simulink model "system2"  (R2020a)
settings: Solver=ode45  StartTime=0.0  StopTime=1  RelTol=1e-3  EnableMultiTasking=on
libraries: powerlib x76, powerlib_meascontrol x8, simulink_extras x8, re_lib x4
settings Model: Creator=srish  LastModifiedBy=srishtik
settings SolverCC: DecoupledContinuousIntegration=on
settings DataIOCC: LimitDataPoints=on  SaveFormat=Array
settings OptimizationCC: LifeSpan=inf
settings DebuggingCC: ReadBeforeWriteMsg=DisableAll  WriteAfterWriteMsg=DisableAll  WriteAfterReadMsg=DisableAll  SolverPrmCheckMsg=warning  MultiTaskDSMMsg=none  SFUnexpectedBacktrackingDiag=warning  SFNoUnconditionalDefaultTransitionDiag=warning  SFExecutionAtInitializationDiag=none  ArithmeticOperatorsInVariantConditions=warning
settings HardwareCC: ProdBitPerPointer=32  ProdBitPerSizeT=32  ProdBitPerPtrDiffT=32  ProdLargestAtomicFloat=None  ProdIntDivRoundTo=Undefined  ProdEndianess=Unspecified  ProdWordSize=32  ProdHWDeviceType=32-bit Generic
settings ModelReferenceCC: UpdateModelReferenceTargets=IfOutOfDate  PropagateSignalLabelsOutOfModel=off
settings SFSimCC: SFSimEcho=off  SimUseLocalCustomCode=off  CustomCodeUndefinedFunction=UseInterfaceOnly
settings RTWCC: RTWUseLocalCustomCode=off
settings CodeAppCC: StateflowObjectComments=on
settings GRTTargetCC: TargetLangStandard=C89/C90 (ANSI)
settings ConfigComp: CovMetricSettings=dw  CovHtmlReporting=on  CovSaveCumulativeToWorkspaceVar=on  CovSaveSingleToWorkspaceVar=on  CovExternalEMLEnable=off  CovSFcnEnable=off
settings SimscapeCC: SimscapeNormalizeSystem=off

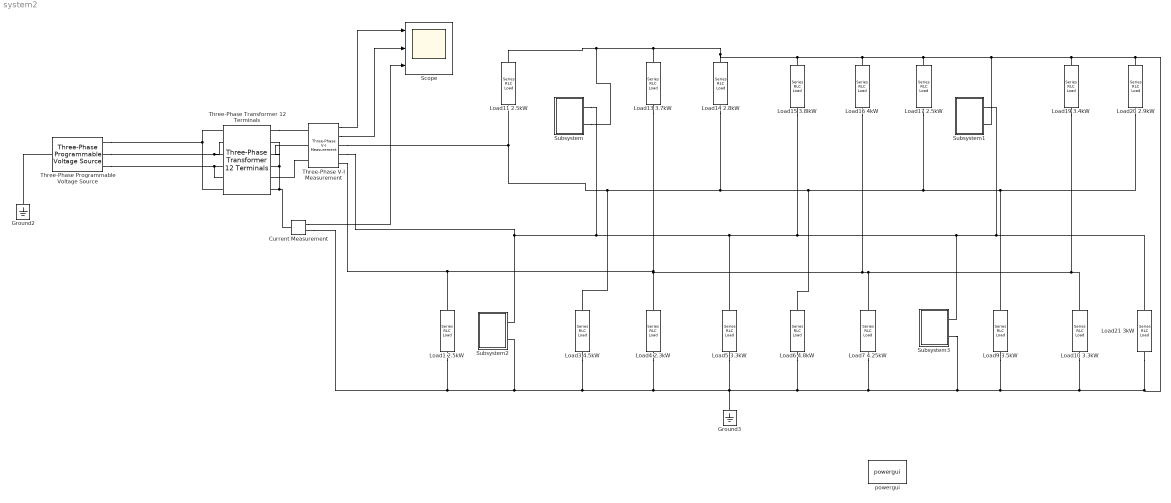
== system system2 ==
  " Load1 2.5kW" : powerlib/Elements/Series RLC Load  LConnTagsString=a  RConnTagsString=__new0  NominalVoltage=254  NominalFrequency=50  ActivePower=2500  InductivePower=1550  CapacitivePower=0  Setx0=off  InitialVoltage=0  SetiL0=off  InitialCurrent=0  Measurements=None  LoadType=constant Z
  " Load10 3.3kW " : powerlib/Elements/Series RLC Load  LConnTagsString=a  RConnTagsString=__new0  NominalVoltage=254  NominalFrequency=50  ActivePower=3300  InductivePower=2046  CapacitivePower=0  Setx0=off  InitialVoltage=0  SetiL0=off  InitialCurrent=0  Measurements=None  LoadType=constant Z
  " Load11 2.5kW" : powerlib/Elements/Series RLC Load  LConnTagsString=a  RConnTagsString=__new0  NominalVoltage=254  NominalFrequency=50  ActivePower=2500  InductivePower=1550  CapacitivePower=0  Setx0=off  InitialVoltage=0  SetiL0=off  InitialCurrent=0  Measurements=None  LoadType=constant Z
  " Load13 3.7kW" : powerlib/Elements/Series RLC Load  LConnTagsString=a  RConnTagsString=__new0  NominalVoltage=254  NominalFrequency=50  ActivePower=3700  InductivePower=2294  CapacitivePower=0  Setx0=off  InitialVoltage=0  SetiL0=off  InitialCurrent=0  Measurements=None  LoadType=constant Z
  " Load14 2.8kW" : powerlib/Elements/Series RLC Load  LConnTagsString=a  RConnTagsString=__new0  NominalVoltage=254  NominalFrequency=50  ActivePower=2800  InductivePower=1736  CapacitivePower=0  Setx0=off  InitialVoltage=0  SetiL0=off  InitialCurrent=0  Measurements=None  LoadType=constant Z
  " Load15 3.8lkW" : powerlib/Elements/Series RLC Load  LConnTagsString=a  RConnTagsString=__new0  NominalVoltage=254  NominalFrequency=50  ActivePower=3800  InductivePower=2356  CapacitivePower=0  Setx0=off  InitialVoltage=0  SetiL0=off  InitialCurrent=0  Measurements=None  LoadType=constant Z
  " Load19 3.4kW" : powerlib/Elements/Series RLC Load  LConnTagsString=a  RConnTagsString=__new0  NominalVoltage=254  NominalFrequency=50  ActivePower=3400  InductivePower=2108  CapacitivePower=0  Setx0=off  InitialVoltage=0  SetiL0=off  InitialCurrent=0  Measurements=None  LoadType=constant Z
  " Load21 3kW" : powerlib/Elements/Series RLC Load  LConnTagsString=a  RConnTagsString=__new0  NominalVoltage=254  NominalFrequency=50  ActivePower=3000  InductivePower=3128  CapacitivePower=0  Setx0=off  InitialVoltage=0  SetiL0=off  InitialCurrent=0  Measurements=None  LoadType=constant Z
  " Load3 4.5kW" : powerlib/Elements/Series RLC Load  LConnTagsString=a  RConnTagsString=__new0  NominalVoltage=254  NominalFrequency=50  ActivePower=4500  InductivePower=2790  CapacitivePower=0  Setx0=off  InitialVoltage=0  SetiL0=off  InitialCurrent=0  Measurements=None  LoadType=constant Z
  " Load4 2.3kW " : powerlib/Elements/Series RLC Load  LConnTagsString=a  RConnTagsString=__new0  NominalVoltage=254  NominalFrequency=50  ActivePower=2300  InductivePower=1426  CapacitivePower=0  Setx0=off  InitialVoltage=0  SetiL0=off  InitialCurrent=0  Measurements=None  LoadType=constant Z
  " Load5 3.3kW" : powerlib/Elements/Series RLC Load  LConnTagsString=a  RConnTagsString=__new0  NominalVoltage=254  NominalFrequency=50  ActivePower=3300  InductivePower=2046  CapacitivePower=0  Setx0=off  InitialVoltage=0  SetiL0=off  InitialCurrent=0  Measurements=None  LoadType=constant Z
  " Load6 4.8kW" : powerlib/Elements/Series RLC Load  LConnTagsString=a  RConnTagsString=__new0  NominalVoltage=254  NominalFrequency=50  ActivePower=4800  InductivePower=2976  CapacitivePower=0  Setx0=off  InitialVoltage=0  SetiL0=off  InitialCurrent=0  Measurements=None  LoadType=constant Z
  " Load7 4.25kW" : powerlib/Elements/Series RLC Load  LConnTagsString=a  RConnTagsString=__new0  NominalVoltage=254  NominalFrequency=50  ActivePower=4250  InductivePower=2635  CapacitivePower=0  Setx0=off  InitialVoltage=0  SetiL0=off  InitialCurrent=0  Measurements=None  LoadType=constant Z
  " Load9 3.5kW" : powerlib/Elements/Series RLC Load  LConnTagsString=a  RConnTagsString=__new0  NominalVoltage=254  NominalFrequency=50  ActivePower=3500  InductivePower=2170  CapacitivePower=0  Setx0=off  InitialVoltage=0  SetiL0=off  InitialCurrent=0  Measurements=None  LoadType=constant Z
  Current Measurement : powerlib/Measurements/Current Measurement  PhasorSimulation=off  OutputType=Complex  PSBequivalent=0
  Ground2 : powerlib/Elements/Ground  LConnTagsString=a
  Ground3 : powerlib/Elements/Ground  LConnTagsString=a
  Load16 4kW : powerlib/Elements/Series RLC Load  LConnTagsString=a  RConnTagsString=__new0  NominalVoltage=254  NominalFrequency=50  ActivePower=4000  InductivePower=2480  CapacitivePower=0  Setx0=off  InitialVoltage=0  SetiL0=off  InitialCurrent=0  Measurements=None  LoadType=constant Z
  Load17 2.5kW : powerlib/Elements/Series RLC Load  LConnTagsString=a  RConnTagsString=__new0  NominalVoltage=254  NominalFrequency=50  ActivePower=2500  InductivePower=1550  CapacitivePower=0  Setx0=off  InitialVoltage=0  SetiL0=off  InitialCurrent=0  Measurements=None  LoadType=constant Z
  Load20 2.9kW : powerlib/Elements/Series RLC Load  LConnTagsString=a  RConnTagsString=__new0  NominalVoltage=254  NominalFrequency=50  ActivePower=2900  InductivePower=1798  CapacitivePower=0  Setx0=off  InitialVoltage=0  SetiL0=off  InitialCurrent=0  Measurements=None  LoadType=constant Z
  Scope : Scope  NumInputPorts=3
  Subsystem : Subsystem
  Subsystem1 : Subsystem
  Subsystem2 : Subsystem
  Subsystem3 : Subsystem
  Three-Phase Programmable Voltage Source : powerlib/Electrical Sources/Three-Phase Programmable Voltage Source  PositiveSequence="[6351  0 50]"  VariationEntity=None  VariationType=Table of time-amplitude pairs  VariationTypeAlt=Step  VariationStep=0.5  VariationRate=10  VariationMagnitude=0.3  VariationFrequency=2  VariationTiming=[1 2]  VariationPhaseA=off  Amplitudes=[1 0.8 1.2 1.0]  TimeValues=[0 0.1 0.15 0.2]  HarmonicGeneration=off  HarmonicA=[3 0.2 -25 0]  HarmonicB=[2 0.15 35 2]  Timing="[0.05  3]"  BusType=swing  Pref=0  Qref=0  Qmin=-inf  Qmax=inf
  Three-Phase V-I Measurement : powerlib/Measurements/Three-Phase V-I Measurement  VoltageMeasurement=phase-to-ground  SetLabelV=off  LabelV=Vabc  Vpu=off  VpuLL=off  CurrentMeasurement=yes  SetLabelI=off  LabelI=Iabc  Ipu=off  Pbase=100e6  Vbase=500e3  OutputType=Complex  PhasorSimulation=off  PSBequivalent=0
  Three-Phase Transformer 12 Terminals : powerlib/Elements/Three-Phase Transformer 12 Terminals  RatedPower=[ 10e6 50 ]  Winding1="[ 6351 0.002  0.05 ]"  Winding2=[ 254 0.002 0.05]  RmXm=[ 200 200 ]
      settings: SourceProductBaseCode=PS
  powergui : powerlib/powergui  Priority=1  SimulationMode=Continuous  SampleTime=50e-6  frequency=60  Iterations=50  frequencyindice=50  Pbase=100e6  ErrMax=1e-4  UnitsV=kV  UnitsW=MW  buscounter=0  FunctionMessages=off  echomessages=off  EnableUseOfTLC=off  CurrentSourceSwitches=on  DisableSnubberDevices=off  DisableRonSwitches=off  DisableVfSwitches=off  DisplayEquations=off  AutomaticDiscreteSolvers=off  SolverType=Tustin  Interpol=off  ExternalGateDelay=off  methode=off  Ts=0  x0status=blocks  SPID=off  SwTol=0  HookPort=off  NonlinearTolerance=1e-4  nMaxIteration=100  ContinueOnMaxIteration=off  RestoreLinks=warning  ResistiveCurrentMeasurement=off  Frange=[0:2:500]  Ylog=off  Xlog=on  ShowGrid=off  save=off  variable=ZData  structure=0  ZoomFFT=off  StartTime=0.0  cycles=1  DisplayStyle=1  fundamental=60  FreqAxis=off  MaxFrequency=1000  frequencyindicesteady=1  RmsSteady=1  display=off
  wires:
  Three-Phase V-I Measurement/1 -> Scope/1
  Three-Phase V-I Measurement/2 -> Scope/2
  Current Measurement/1 -> Scope/3
  connections:
  " Load3 4.5kW"/RConn1 -- " Load4 2.3kW "/RConn1 -- " Load5 3.3kW"/RConn1 -- " Load6 4.8kW"/RConn1 -- Subsystem3/RConn2 -- " Load9 3.5kW"/RConn1 -- " Load10 3.3kW "/RConn1 -- " Load21 3kW"/RConn1 -- Subsystem1/RConn2 -- Subsystem/RConn2 -- " Load11 2.5kW"/LConn1 -- " Load13 3.7kW"/LConn1 -- " Load14 2.8kW"/LConn1 -- " Load15 3.8lkW"/LConn1 -- Load16 4kW/LConn1 -- Load17 2.5kW/LConn1 -- " Load19 3.4kW"/LConn1 -- Load20 2.9kW/LConn1 -- " Load7 4.25kW"/RConn1 -- Ground3/LConn1 -- Subsystem2/RConn2 -- Current Measurement/RConn1 -- " Load1 2.5kW"/RConn1
  Three-Phase Transformer 12 Terminals/RConn1 -- Three-Phase V-I Measurement/LConn1
  Three-Phase Transformer 12 Terminals/RConn3 -- Three-Phase V-I Measurement/LConn2
  Three-Phase Transformer 12 Terminals/RConn5 -- Three-Phase V-I Measurement/LConn3
  Three-Phase V-I Measurement/RConn3 -- Load16 4kW/RConn1 -- " Load19 3.4kW"/RConn1 -- " Load10 3.3kW "/LConn1 -- " Load7 4.25kW"/LConn1 -- " Load4 2.3kW "/LConn1 -- " Load13 3.7kW"/RConn1 -- " Load1 2.5kW"/LConn1
  Three-Phase V-I Measurement/RConn2 -- Subsystem2/RConn1 -- Subsystem/RConn1 -- Subsystem3/RConn1 -- " Load21 3kW"/LConn1 -- Subsystem1/RConn1 -- " Load15 3.8lkW"/RConn1 -- " Load5 3.3kW"/LConn1
  Three-Phase V-I Measurement/RConn1 -- " Load3 4.5kW"/LConn1 -- " Load6 4.8kW"/LConn1 -- Load20 2.9kW/RConn1 -- " Load9 3.5kW"/LConn1 -- Load17 2.5kW/RConn1 -- " Load14 2.8kW"/RConn1 -- " Load11 2.5kW"/RConn1
  Three-Phase Programmable Voltage Source/LConn1 -- Ground2/LConn1
  Three-Phase Programmable Voltage Source/RConn1 -- Three-Phase Transformer 12 Terminals/LConn1 -- Three-Phase Transformer 12 Terminals/LConn6
  Three-Phase Transformer 12 Terminals/LConn3 -- Three-Phase Transformer 12 Terminals/LConn2 -- Three-Phase Programmable Voltage Source/RConn2
  Three-Phase Transformer 12 Terminals/LConn4 -- Three-Phase Transformer 12 Terminals/LConn5 -- Three-Phase Programmable Voltage Source/RConn3
  Current Measurement/LConn1 -- Three-Phase Transformer 12 Terminals/RConn2 -- Three-Phase Transformer 12 Terminals/RConn4 -- Three-Phase Transformer 12 Terminals/RConn6

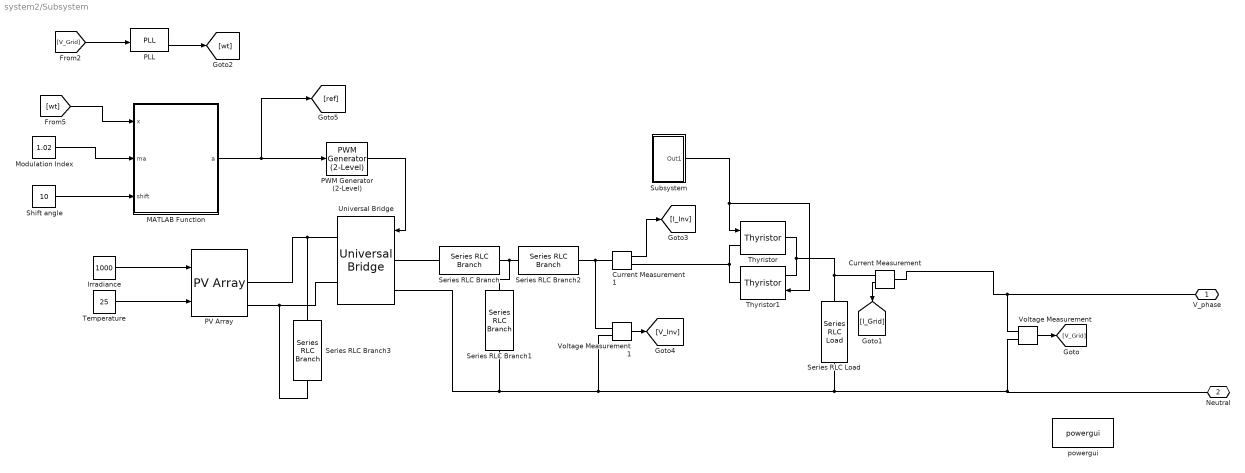
== system system2/Subsystem ==
  Current Measurement : powerlib/Measurements/Current Measurement  PhasorSimulation=off  OutputType=Complex  PSBequivalent=0
  Current Measurement1 : powerlib/Measurements/Current Measurement  PhasorSimulation=off  OutputType=Complex  PSBequivalent=0
  Irradiance : Constant  Value=1000
  MATLAB Function : MATLAB Function  TreatAsAtomicUnit=on
  Modulation Index : Constant  Value=1.02
  PLL : powerlib_meascontrol/PLL/PLL  Fmin=45  Par_Init=[0, 50]  ParK=[180, 3200, 1]  TcD=1e-4  MaxRateChangeFreq=12  FilterCutOffFreq=25  Ts=1e-04  AGC=on
      settings: SourceProductBaseCode=PS
  PV Array : re_lib/Solar/PV Array  Npar=10  Nser=12  PlotType=array @ 1000 W/m2 & specified temperatures  S_vec="[ 1000  500  100 ]"  Temp_C_vec="[ 45 25  ]"  ModuleName=1Soltech 1STH-215-P  PlotWhenSelected=off  Pm=213.15  Ncell=60  Voc=36.3  Isc=7.84  Vm=29  Im=7.35  beta_Voc_pc=-0.36099  alpha_Isc_pc=0.102  beta_Voc=-0.13104  alpha_Isc=0.007997  IL=7.8649  I0=2.9259e-10  nI=0.98117  Rsh=313.3991  Rs=0.39383  RobustModel=off  RobustCellTemperature=25  BAL=off  Tc=1e-6  Tfilter=5e-5
  PWM Generator (2-Level) : powerlib_meascontrol/Pulse & Signal Generators/PWM Generator (2-Level)  ModulatorType=Single-phase full-bridge (4 pulses)  ModulatorMode=Unsynchronized  Fc=5000  Pc=0  nF=27  MinMax="[ -1  1 ]"  SamplingTechnique=Natural  ModulatingSignals=off  m=0.8  Freq=60  Phase=0  Ts=0  ShowCarrierOutport=off
  Series RLC Branch : powerlib/Elements/Series RLC Branch  LConnTagsString=__new0  RConnTagsString=__new0  BranchType=L  Resistance=1  Inductance=12.96e-03  SetiL0=off  InitialCurrent=0  Capacitance=1e-6  Setx0=off  InitialVoltage=0  Measurements=None
  Series RLC Branch1 : powerlib/Elements/Series RLC Branch  LConnTagsString=__new0  RConnTagsString=__new0  BranchType=RC  Resistance=2  Inductance=8.59e-04  SetiL0=off  InitialCurrent=0  Capacitance=12.33e-06  Setx0=off  InitialVoltage=0  Measurements=None
  Series RLC Branch2 : powerlib/Elements/Series RLC Branch  LConnTagsString=__new0  RConnTagsString=__new0  BranchType=L  Resistance=1  Inductance=0.45e-03  SetiL0=off  InitialCurrent=0  Capacitance=1e-6  Setx0=off  InitialVoltage=0  Measurements=None
  Series RLC Branch3 : powerlib/Elements/Series RLC Branch  LConnTagsString=__new0  RConnTagsString=__new0  BranchType=C  Resistance=2  Inductance=8.59e-04  SetiL0=off  InitialCurrent=0  Capacitance=1000e-06  Setx0=off  InitialVoltage=0  Measurements=None
  Series RLC Load : powerlib/Elements/Series RLC Load  LConnTagsString=a  RConnTagsString=__new0  NominalVoltage=254  NominalFrequency=50  ActivePower=5000  InductivePower=3100  CapacitivePower=0  Setx0=off  InitialVoltage=0  SetiL0=off  InitialCurrent=0  Measurements=None  LoadType=constant Z
  "Shift angle " : Constant  Value=10
  Subsystem : Subsystem
  "Temperature " : Constant  Value=25
  Thyristor : powerlib/Power Electronics/Thyristor  Ron=0.001  Lon=0  Vf=0.8  IC=0  Rs=500  Cs=250e-9  Measurements=off
  Thyristor1 : powerlib/Power Electronics/Thyristor  Ron=0.001  Lon=0  Vf=0.8  IC=0  Rs=500  Cs=250e-9  Measurements=off
  Universal Bridge : powerlib/Power Electronics/Universal Bridge  Arms=2  SnubberResistance=1e5  SnubberCapacitance=inf  Device=IGBT / Diodes  Ron=1e-3  Lon=0  ForwardVoltages="[  0  0  ]"  ForwardVoltage=0  GTOparameters=[ 10e-6 , 20e-6 ]  IGBTparameters=[ 1e-6 , 2e-6 ]  Measurements=None  Measurements_2=None  converterType=Rectifier
  Voltage Measurement : powerlib/Measurements/Voltage Measurement  PhasorSimulation=off  OutputType=Complex  PSBequivalent=0
  Voltage Measurement1 : powerlib/Measurements/Voltage Measurement  PhasorSimulation=off  OutputType=Complex  PSBequivalent=0
  powergui : powerlib/powergui  Priority=1  SimulationMode=Continuous  SampleTime=50e-6  frequency=60  Iterations=50  frequencyindice=0  Pbase=100e6  ErrMax=1e-4  UnitsV=kV  UnitsW=MW  buscounter=0  FunctionMessages=off  echomessages=off  EnableUseOfTLC=off  CurrentSourceSwitches=off  DisableSnubberDevices=off  DisableRonSwitches=off  DisableVfSwitches=off  DisplayEquations=off  AutomaticDiscreteSolvers=off  SolverType=Tustin/Backward Euler (TBE)  Interpol=off  ExternalGateDelay=off  methode=off  Ts=100  x0status=blocks  SPID=on  SwTol=0  HookPort=off  NonlinearTolerance=1e-4  nMaxIteration=100  ContinueOnMaxIteration=off  RestoreLinks=warning  ResistiveCurrentMeasurement=off  Frange=[0:2:500]  Ylog=off  Xlog=on  ShowGrid=off  save=off  variable=ZData  structure=0  ZoomFFT=off  StartTime=0.0  cycles=1  DisplayStyle=1  fundamental=60  FreqAxis=off  MaxFrequency=1000  frequencyindicesteady=1  RmsSteady=1  display=off
  V_phase : PMIOPort  Side=Right
  "Neutral " : PMIOPort  Port=2  Side=Right
  wires:
  MATLAB Function/1(a) -> [ref], PWM Generator (2-Level)/1
  Current Measurement/1 -> [I_Grid]
  Voltage Measurement/1 -> [V_Grid]
  "Shift angle "/1 -> MATLAB Function/3(shift)
  PWM Generator (2-Level)/1 -> Universal Bridge/1
  Voltage Measurement1/1 -> [V_Inv]
  Modulation Index/1 -> MATLAB Function/2(ma)
  [V_Grid] -> PLL/1
  PLL/2 -> [wt]
  [wt] -> MATLAB Function/1(x)
  Irradiance/1 -> PV Array/1
  "Temperature "/1 -> PV Array/2
  Current Measurement1/1 -> [I_Inv]
  Subsystem/1(Out1) -> Thyristor1/1, Thyristor/1
  connections:
  Thyristor/RConn1 -- Series RLC Load/LConn1 -- Current Measurement/RConn1 -- Thyristor1/LConn1
  Universal Bridge/LConn2 -- Series RLC Branch1/RConn1 -- Voltage Measurement1/LConn2 -- "Neutral "/RConn1 -- Voltage Measurement/LConn2 -- Series RLC Load/RConn1
  Series RLC Branch/RConn1 -- Series RLC Branch2/LConn1 -- Series RLC Branch1/LConn1
  Current Measurement/LConn1 -- V_phase/RConn1 -- Voltage Measurement/LConn1
  Universal Bridge/LConn1 -- Series RLC Branch/LConn1
  Series RLC Branch2/RConn1 -- Voltage Measurement1/LConn1 -- Current Measurement1/LConn1
  PV Array/RConn1 -- Universal Bridge/RConn1 -- Series RLC Branch3/LConn1
  PV Array/RConn2 -- Series RLC Branch3/RConn1 -- Universal Bridge/RConn2
  Thyristor/LConn1 -- Current Measurement1/RConn1 -- Thyristor1/RConn1

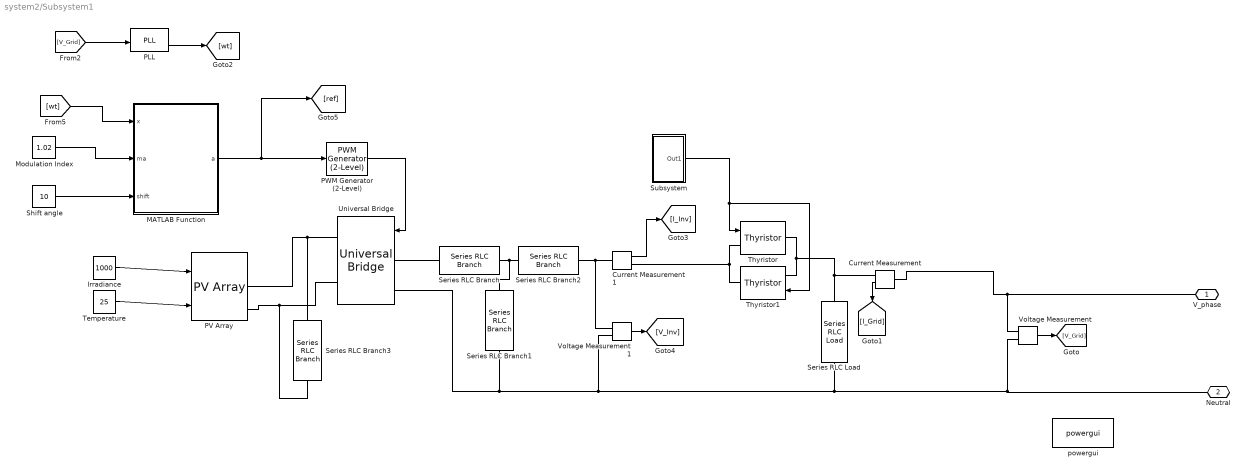
== system system2/Subsystem1 ==
  Current Measurement : powerlib/Measurements/Current Measurement  PhasorSimulation=off  OutputType=Complex  PSBequivalent=0
  Current Measurement1 : powerlib/Measurements/Current Measurement  PhasorSimulation=off  OutputType=Complex  PSBequivalent=0
  Irradiance : Constant  Value=1000
  MATLAB Function : MATLAB Function  TreatAsAtomicUnit=on
  Modulation Index : Constant  Value=1.02
  PLL : powerlib_meascontrol/PLL/PLL  Fmin=45  Par_Init=[0, 50]  ParK=[180, 3200, 1]  TcD=1e-4  MaxRateChangeFreq=12  FilterCutOffFreq=25  Ts=1e-04  AGC=on
      settings: SourceProductBaseCode=PS
  PV Array : re_lib/Solar/PV Array  Npar=10  Nser=12  PlotType=array @ 1000 W/m2 & specified temperatures  S_vec="[ 1000  500  100 ]"  Temp_C_vec="[ 45 25  ]"  ModuleName=1Soltech 1STH-215-P  PlotWhenSelected=off  Pm=213.15  Ncell=60  Voc=36.3  Isc=7.84  Vm=29  Im=7.35  beta_Voc_pc=-0.36099  alpha_Isc_pc=0.102  beta_Voc=-0.13104  alpha_Isc=0.007997  IL=7.8649  I0=2.9259e-10  nI=0.98117  Rsh=313.3991  Rs=0.39383  RobustModel=off  RobustCellTemperature=25  BAL=off  Tc=1e-6  Tfilter=5e-5
  PWM Generator (2-Level) : powerlib_meascontrol/Pulse & Signal Generators/PWM Generator (2-Level)  ModulatorType=Single-phase full-bridge (4 pulses)  ModulatorMode=Unsynchronized  Fc=5000  Pc=0  nF=27  MinMax="[ -1  1 ]"  SamplingTechnique=Natural  ModulatingSignals=off  m=0.8  Freq=60  Phase=0  Ts=0  ShowCarrierOutport=off
  Series RLC Branch : powerlib/Elements/Series RLC Branch  LConnTagsString=__new0  RConnTagsString=__new0  BranchType=L  Resistance=1  Inductance=12.96e-03  SetiL0=off  InitialCurrent=0  Capacitance=1e-6  Setx0=off  InitialVoltage=0  Measurements=None
  Series RLC Branch1 : powerlib/Elements/Series RLC Branch  LConnTagsString=__new0  RConnTagsString=__new0  BranchType=RC  Resistance=2  Inductance=8.59e-04  SetiL0=off  InitialCurrent=0  Capacitance=12.33e-06  Setx0=off  InitialVoltage=0  Measurements=None
  Series RLC Branch2 : powerlib/Elements/Series RLC Branch  LConnTagsString=__new0  RConnTagsString=__new0  BranchType=L  Resistance=1  Inductance=0.45e-03  SetiL0=off  InitialCurrent=0  Capacitance=1e-6  Setx0=off  InitialVoltage=0  Measurements=None
  Series RLC Branch3 : powerlib/Elements/Series RLC Branch  LConnTagsString=__new0  RConnTagsString=__new0  BranchType=C  Resistance=2  Inductance=8.59e-04  SetiL0=off  InitialCurrent=0  Capacitance=1000e-06  Setx0=off  InitialVoltage=0  Measurements=None
  Series RLC Load : powerlib/Elements/Series RLC Load  LConnTagsString=a  RConnTagsString=__new0  NominalVoltage=254  NominalFrequency=50  ActivePower=4900  InductivePower=3038  CapacitivePower=0  Setx0=off  InitialVoltage=0  SetiL0=off  InitialCurrent=0  Measurements=None  LoadType=constant Z
  "Shift angle " : Constant  Value=10
  Subsystem : Subsystem
  "Temperature " : Constant  Value=25
  Thyristor : powerlib/Power Electronics/Thyristor  Ron=0.001  Lon=0  Vf=0.8  IC=0  Rs=500  Cs=250e-9  Measurements=off
  Thyristor1 : powerlib/Power Electronics/Thyristor  Ron=0.001  Lon=0  Vf=0.8  IC=0  Rs=500  Cs=250e-9  Measurements=off
  Universal Bridge : powerlib/Power Electronics/Universal Bridge  Arms=2  SnubberResistance=1e5  SnubberCapacitance=inf  Device=IGBT / Diodes  Ron=1e-3  Lon=0  ForwardVoltages="[  0  0  ]"  ForwardVoltage=0  GTOparameters=[ 10e-6 , 20e-6 ]  IGBTparameters=[ 1e-6 , 2e-6 ]  Measurements=None  Measurements_2=None  converterType=Rectifier
  Voltage Measurement : powerlib/Measurements/Voltage Measurement  PhasorSimulation=off  OutputType=Complex  PSBequivalent=0
  Voltage Measurement1 : powerlib/Measurements/Voltage Measurement  PhasorSimulation=off  OutputType=Complex  PSBequivalent=0
  powergui : powerlib/powergui  Priority=1  SimulationMode=Continuous  SampleTime=50e-6  frequency=60  Iterations=50  frequencyindice=0  Pbase=100e6  ErrMax=1e-4  UnitsV=kV  UnitsW=MW  buscounter=0  FunctionMessages=off  echomessages=off  EnableUseOfTLC=off  CurrentSourceSwitches=off  DisableSnubberDevices=off  DisableRonSwitches=off  DisableVfSwitches=off  DisplayEquations=off  AutomaticDiscreteSolvers=off  SolverType=Tustin/Backward Euler (TBE)  Interpol=off  ExternalGateDelay=off  methode=off  Ts=100  x0status=blocks  SPID=on  SwTol=0  HookPort=off  NonlinearTolerance=1e-4  nMaxIteration=100  ContinueOnMaxIteration=off  RestoreLinks=warning  ResistiveCurrentMeasurement=off  Frange=[0:2:500]  Ylog=off  Xlog=on  ShowGrid=off  save=off  variable=ZData  structure=0  ZoomFFT=off  StartTime=0.0  cycles=1  DisplayStyle=1  fundamental=60  FreqAxis=off  MaxFrequency=1000  frequencyindicesteady=1  RmsSteady=1  display=off
  V_phase : PMIOPort  Side=Right
  "Neutral " : PMIOPort  Port=2  Side=Right
  wires:
  Subsystem/1(Out1) -> Thyristor/1, Thyristor1/1
  Current Measurement1/1 -> [I_Inv]
  "Temperature "/1 -> PV Array/2
  Irradiance/1 -> PV Array/1
  [wt] -> MATLAB Function/1(x)
  PLL/2 -> [wt]
  [V_Grid] -> PLL/1
  Modulation Index/1 -> MATLAB Function/2(ma)
  Voltage Measurement1/1 -> [V_Inv]
  PWM Generator (2-Level)/1 -> Universal Bridge/1
  "Shift angle "/1 -> MATLAB Function/3(shift)
  Voltage Measurement/1 -> [V_Grid]
  Current Measurement/1 -> [I_Grid]
  MATLAB Function/1(a) -> PWM Generator (2-Level)/1, [ref]
  connections:
  Thyristor1/RConn1 -- Current Measurement1/RConn1 -- Thyristor/LConn1
  Universal Bridge/RConn2 -- Series RLC Branch3/RConn1 -- PV Array/RConn2
  Series RLC Branch3/LConn1 -- Universal Bridge/RConn1 -- PV Array/RConn1
  Current Measurement1/LConn1 -- Voltage Measurement1/LConn1 -- Series RLC Branch2/RConn1
  Universal Bridge/LConn1 -- Series RLC Branch/LConn1
  Voltage Measurement/LConn1 -- V_phase/RConn1 -- Current Measurement/LConn1
  Series RLC Branch1/LConn1 -- Series RLC Branch2/LConn1 -- Series RLC Branch/RConn1
  Series RLC Load/RConn1 -- Voltage Measurement/LConn2 -- "Neutral "/RConn1 -- Voltage Measurement1/LConn2 -- Series RLC Branch1/RConn1 -- Universal Bridge/LConn2
  Thyristor1/LConn1 -- Current Measurement/RConn1 -- Series RLC Load/LConn1 -- Thyristor/RConn1

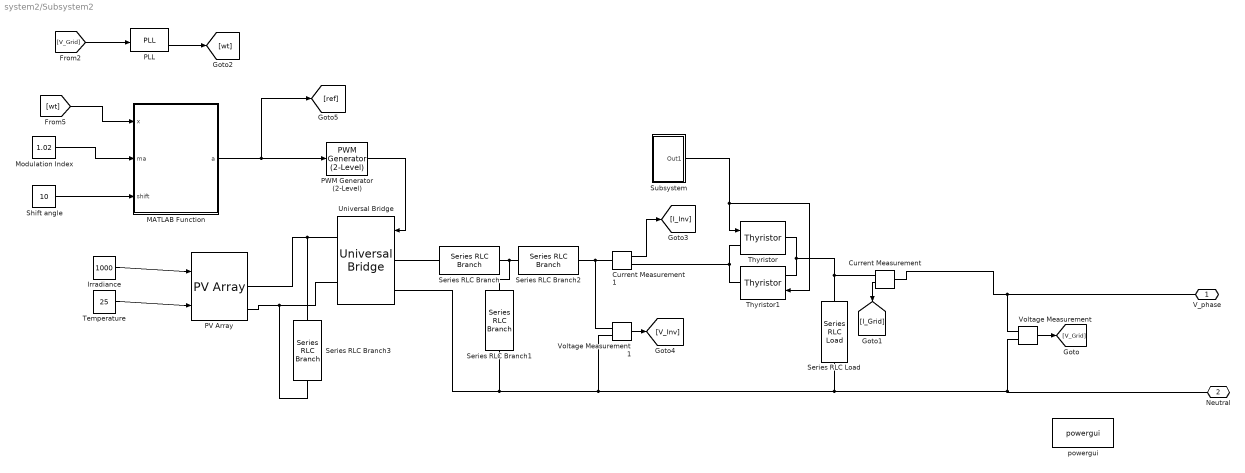
== system system2/Subsystem2 ==
  Current Measurement : powerlib/Measurements/Current Measurement  PhasorSimulation=off  OutputType=Complex  PSBequivalent=0
  Current Measurement1 : powerlib/Measurements/Current Measurement  PhasorSimulation=off  OutputType=Complex  PSBequivalent=0
  Irradiance : Constant  Value=1000
  MATLAB Function : MATLAB Function  TreatAsAtomicUnit=on
  Modulation Index : Constant  Value=1.02
  PLL : powerlib_meascontrol/PLL/PLL  Fmin=45  Par_Init=[0, 50]  ParK=[180, 3200, 1]  TcD=1e-4  MaxRateChangeFreq=12  FilterCutOffFreq=25  Ts=1e-04  AGC=on
      settings: SourceProductBaseCode=PS
  PV Array : re_lib/Solar/PV Array  Npar=10  Nser=12  PlotType=array @ 1000 W/m2 & specified temperatures  S_vec="[ 1000  500  100 ]"  Temp_C_vec="[ 45 25  ]"  ModuleName=1Soltech 1STH-215-P  PlotWhenSelected=off  Pm=213.15  Ncell=60  Voc=36.3  Isc=7.84  Vm=29  Im=7.35  beta_Voc_pc=-0.36099  alpha_Isc_pc=0.102  beta_Voc=-0.13104  alpha_Isc=0.007997  IL=7.8649  I0=2.9259e-10  nI=0.98117  Rsh=313.3991  Rs=0.39383  RobustModel=off  RobustCellTemperature=25  BAL=off  Tc=1e-6  Tfilter=5e-5
  PWM Generator (2-Level) : powerlib_meascontrol/Pulse & Signal Generators/PWM Generator (2-Level)  ModulatorType=Single-phase full-bridge (4 pulses)  ModulatorMode=Unsynchronized  Fc=5000  Pc=0  nF=27  MinMax="[ -1  1 ]"  SamplingTechnique=Natural  ModulatingSignals=off  m=0.8  Freq=60  Phase=0  Ts=0  ShowCarrierOutport=off
  Series RLC Branch : powerlib/Elements/Series RLC Branch  LConnTagsString=__new0  RConnTagsString=__new0  BranchType=L  Resistance=1  Inductance=12.96e-03  SetiL0=off  InitialCurrent=0  Capacitance=1e-6  Setx0=off  InitialVoltage=0  Measurements=None
  Series RLC Branch1 : powerlib/Elements/Series RLC Branch  LConnTagsString=__new0  RConnTagsString=__new0  BranchType=RC  Resistance=2  Inductance=8.59e-04  SetiL0=off  InitialCurrent=0  Capacitance=12.33e-06  Setx0=off  InitialVoltage=0  Measurements=None
  Series RLC Branch2 : powerlib/Elements/Series RLC Branch  LConnTagsString=__new0  RConnTagsString=__new0  BranchType=L  Resistance=1  Inductance=0.45e-03  SetiL0=off  InitialCurrent=0  Capacitance=1e-6  Setx0=off  InitialVoltage=0  Measurements=None
  Series RLC Branch3 : powerlib/Elements/Series RLC Branch  LConnTagsString=__new0  RConnTagsString=__new0  BranchType=C  Resistance=2  Inductance=8.59e-04  SetiL0=off  InitialCurrent=0  Capacitance=1000e-06  Setx0=off  InitialVoltage=0  Measurements=None
  Series RLC Load : powerlib/Elements/Series RLC Load  LConnTagsString=a  RConnTagsString=__new0  NominalVoltage=254  NominalFrequency=50  ActivePower=5000  InductivePower=3100  CapacitivePower=0  Setx0=off  InitialVoltage=0  SetiL0=off  InitialCurrent=0  Measurements=None  LoadType=constant Z
  "Shift angle " : Constant  Value=10
  Subsystem : Subsystem
  "Temperature " : Constant  Value=25
  Thyristor : powerlib/Power Electronics/Thyristor  Ron=0.001  Lon=0  Vf=0.8  IC=0  Rs=500  Cs=250e-9  Measurements=off
  Thyristor1 : powerlib/Power Electronics/Thyristor  Ron=0.001  Lon=0  Vf=0.8  IC=0  Rs=500  Cs=250e-9  Measurements=off
  Universal Bridge : powerlib/Power Electronics/Universal Bridge  Arms=2  SnubberResistance=1e5  SnubberCapacitance=inf  Device=IGBT / Diodes  Ron=1e-3  Lon=0  ForwardVoltages="[  0  0  ]"  ForwardVoltage=0  GTOparameters=[ 10e-6 , 20e-6 ]  IGBTparameters=[ 1e-6 , 2e-6 ]  Measurements=None  Measurements_2=None  converterType=Rectifier
  Voltage Measurement : powerlib/Measurements/Voltage Measurement  PhasorSimulation=off  OutputType=Complex  PSBequivalent=0
  Voltage Measurement1 : powerlib/Measurements/Voltage Measurement  PhasorSimulation=off  OutputType=Complex  PSBequivalent=0
  powergui : powerlib/powergui  Priority=1  SimulationMode=Continuous  SampleTime=50e-6  frequency=60  Iterations=50  frequencyindice=0  Pbase=100e6  ErrMax=1e-4  UnitsV=kV  UnitsW=MW  buscounter=0  FunctionMessages=off  echomessages=off  EnableUseOfTLC=off  CurrentSourceSwitches=off  DisableSnubberDevices=off  DisableRonSwitches=off  DisableVfSwitches=off  DisplayEquations=off  AutomaticDiscreteSolvers=off  SolverType=Tustin/Backward Euler (TBE)  Interpol=off  ExternalGateDelay=off  methode=off  Ts=100  x0status=blocks  SPID=on  SwTol=0  HookPort=off  NonlinearTolerance=1e-4  nMaxIteration=100  ContinueOnMaxIteration=off  RestoreLinks=warning  ResistiveCurrentMeasurement=off  Frange=[0:2:500]  Ylog=off  Xlog=on  ShowGrid=off  save=off  variable=ZData  structure=0  ZoomFFT=off  StartTime=0.0  cycles=1  DisplayStyle=1  fundamental=60  FreqAxis=off  MaxFrequency=1000  frequencyindicesteady=1  RmsSteady=1  display=off
  V_phase : PMIOPort  Side=Right
  "Neutral " : PMIOPort  Port=2  Side=Right
  wires:
  Subsystem/1(Out1) -> Thyristor/1, Thyristor1/1
  Current Measurement1/1 -> [I_Inv]
  "Temperature "/1 -> PV Array/2
  Irradiance/1 -> PV Array/1
  [wt] -> MATLAB Function/1(x)
  PLL/2 -> [wt]
  [V_Grid] -> PLL/1
  Modulation Index/1 -> MATLAB Function/2(ma)
  Voltage Measurement1/1 -> [V_Inv]
  PWM Generator (2-Level)/1 -> Universal Bridge/1
  "Shift angle "/1 -> MATLAB Function/3(shift)
  Voltage Measurement/1 -> [V_Grid]
  Current Measurement/1 -> [I_Grid]
  MATLAB Function/1(a) -> PWM Generator (2-Level)/1, [ref]
  connections:
  Thyristor1/RConn1 -- Current Measurement1/RConn1 -- Thyristor/LConn1
  Universal Bridge/RConn2 -- Series RLC Branch3/RConn1 -- PV Array/RConn2
  Series RLC Branch3/LConn1 -- Universal Bridge/RConn1 -- PV Array/RConn1
  Current Measurement1/LConn1 -- Voltage Measurement1/LConn1 -- Series RLC Branch2/RConn1
  Universal Bridge/LConn1 -- Series RLC Branch/LConn1
  Voltage Measurement/LConn1 -- V_phase/RConn1 -- Current Measurement/LConn1
  Series RLC Branch1/LConn1 -- Series RLC Branch2/LConn1 -- Series RLC Branch/RConn1
  Series RLC Load/RConn1 -- Voltage Measurement/LConn2 -- "Neutral "/RConn1 -- Voltage Measurement1/LConn2 -- Series RLC Branch1/RConn1 -- Universal Bridge/LConn2
  Thyristor1/LConn1 -- Current Measurement/RConn1 -- Series RLC Load/LConn1 -- Thyristor/RConn1

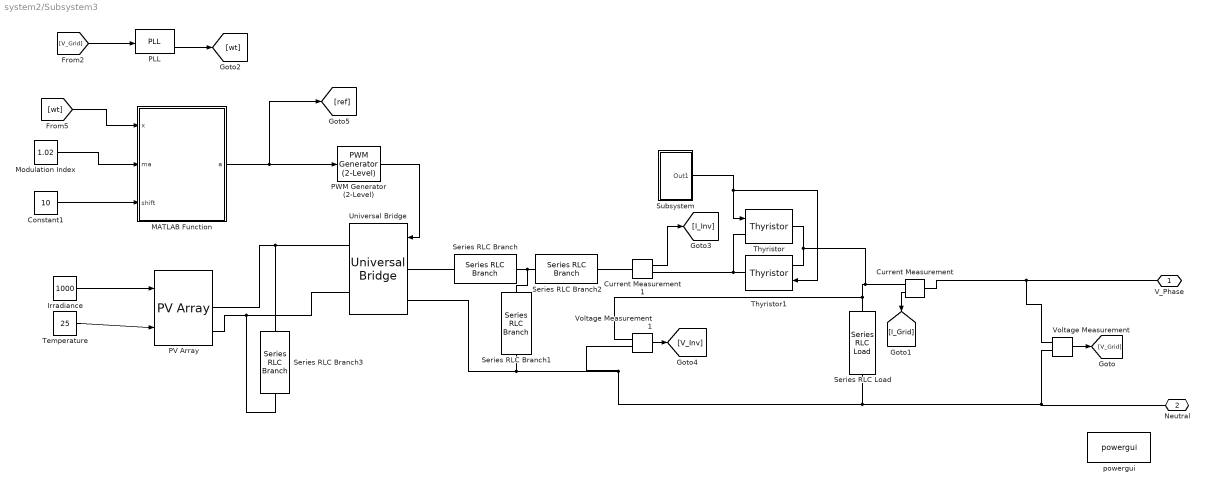
== system system2/Subsystem3 ==
  Constant1 : Constant  Value=10
  Current Measurement : powerlib/Measurements/Current Measurement  PhasorSimulation=off  OutputType=Complex  PSBequivalent=0
  Current Measurement1 : powerlib/Measurements/Current Measurement  PhasorSimulation=off  OutputType=Complex  PSBequivalent=0
  Irradiance : Constant  Value=1000
  MATLAB Function : MATLAB Function  TreatAsAtomicUnit=on
  Modulation Index : Constant  Value=1.02
  PLL : powerlib_meascontrol/PLL/PLL  Fmin=45  Par_Init=[0, 50]  ParK=[180, 3200, 1]  TcD=1e-4  MaxRateChangeFreq=12  FilterCutOffFreq=25  Ts=1e-04  AGC=on
      settings: SourceProductBaseCode=PS
  PV Array : re_lib/Solar/PV Array  Npar=2  Nser=12  PlotType=array @ 1000 W/m2 & specified temperatures  S_vec="[ 1000  500  100 ]"  Temp_C_vec="[ 45 25  ]"  ModuleName=1Soltech 1STH-215-P  PlotWhenSelected=off  Pm=213.15  Ncell=60  Voc=36.3  Isc=7.84  Vm=29  Im=7.35  beta_Voc_pc=-0.36099  alpha_Isc_pc=0.102  beta_Voc=-0.13104  alpha_Isc=0.007997  IL=7.8649  I0=2.9259e-10  nI=0.98117  Rsh=313.3991  Rs=0.39383  RobustModel=off  RobustCellTemperature=25  BAL=off  Tc=1e-6  Tfilter=5e-5
  PWM Generator (2-Level) : powerlib_meascontrol/Pulse & Signal Generators/PWM Generator (2-Level)  ModulatorType=Single-phase full-bridge (4 pulses)  ModulatorMode=Unsynchronized  Fc=5000  Pc=0  nF=27  MinMax="[ -1  1 ]"  SamplingTechnique=Natural  ModulatingSignals=off  m=0.8  Freq=60  Phase=0  Ts=0  ShowCarrierOutport=off
  Series RLC Branch : powerlib/Elements/Series RLC Branch  LConnTagsString=__new0  RConnTagsString=__new0  BranchType=L  Resistance=1  Inductance=12.96e-03  SetiL0=off  InitialCurrent=0  Capacitance=1e-6  Setx0=off  InitialVoltage=0  Measurements=None
  Series RLC Branch1 : powerlib/Elements/Series RLC Branch  LConnTagsString=__new0  RConnTagsString=__new0  BranchType=RC  Resistance=2  Inductance=8.59e-04  SetiL0=off  InitialCurrent=0  Capacitance=12.33e-06  Setx0=off  InitialVoltage=0  Measurements=None
  Series RLC Branch2 : powerlib/Elements/Series RLC Branch  LConnTagsString=__new0  RConnTagsString=__new0  BranchType=L  Resistance=1  Inductance=0.45e-03  SetiL0=off  InitialCurrent=0  Capacitance=1e-6  Setx0=off  InitialVoltage=0  Measurements=None
  Series RLC Branch3 : powerlib/Elements/Series RLC Branch  LConnTagsString=__new0  RConnTagsString=__new0  BranchType=C  Resistance=2  Inductance=8.59e-04  SetiL0=off  InitialCurrent=0  Capacitance=1000e-06  Setx0=off  InitialVoltage=0  Measurements=None
  Series RLC Load : powerlib/Elements/Series RLC Load  LConnTagsString=a  RConnTagsString=__new0  NominalVoltage=254  NominalFrequency=50  ActivePower=2500  InductivePower=1550  CapacitivePower=0  Setx0=off  InitialVoltage=0  SetiL0=off  InitialCurrent=0  Measurements=None  LoadType=constant Z
  Subsystem : Subsystem
  "Temperature " : Constant  Value=25
  Thyristor : powerlib/Power Electronics/Thyristor  Ron=0.001  Lon=0  Vf=0.8  IC=0  Rs=500  Cs=250e-9  Measurements=off
  Thyristor1 : powerlib/Power Electronics/Thyristor  Ron=0.001  Lon=0  Vf=0.8  IC=0  Rs=500  Cs=250e-9  Measurements=off
  Universal Bridge : powerlib/Power Electronics/Universal Bridge  Arms=2  SnubberResistance=1e5  SnubberCapacitance=inf  Device=IGBT / Diodes  Ron=1e-3  Lon=0  ForwardVoltages="[  0  0  ]"  ForwardVoltage=0  GTOparameters=[ 10e-6 , 20e-6 ]  IGBTparameters=[ 1e-6 , 2e-6 ]  Measurements=None  Measurements_2=None  converterType=Rectifier
  Voltage Measurement : powerlib/Measurements/Voltage Measurement  PhasorSimulation=off  OutputType=Complex  PSBequivalent=0
  Voltage Measurement1 : powerlib/Measurements/Voltage Measurement  PhasorSimulation=off  OutputType=Complex  PSBequivalent=0
  powergui : powerlib/powergui  Priority=1  SimulationMode=Continuous  SampleTime=50e-6  frequency=60  Iterations=50  frequencyindice=0  Pbase=100e6  ErrMax=1e-4  UnitsV=kV  UnitsW=MW  buscounter=0  FunctionMessages=off  echomessages=off  EnableUseOfTLC=off  CurrentSourceSwitches=off  DisableSnubberDevices=off  DisableRonSwitches=off  DisableVfSwitches=off  DisplayEquations=off  AutomaticDiscreteSolvers=off  SolverType=Tustin/Backward Euler (TBE)  Interpol=off  ExternalGateDelay=off  methode=off  Ts=100  x0status=blocks  SPID=on  SwTol=0  HookPort=off  NonlinearTolerance=1e-4  nMaxIteration=100  ContinueOnMaxIteration=off  RestoreLinks=warning  ResistiveCurrentMeasurement=off  Frange=[0:2:500]  Ylog=off  Xlog=on  ShowGrid=off  save=off  variable=ZData  structure=0  ZoomFFT=off  StartTime=0.0  cycles=1  DisplayStyle=1  fundamental=60  FreqAxis=off  MaxFrequency=1000  frequencyindicesteady=1  RmsSteady=1  display=off
  V_Phase : PMIOPort  Side=Right
  "Neutral " : PMIOPort  Port=2  Side=Right
  wires:
  MATLAB Function/1(a) -> [ref], PWM Generator (2-Level)/1
  Subsystem/1(Out1) -> Thyristor/1, Thyristor1/1
  Voltage Measurement/1 -> [V_Grid]
  [wt] -> MATLAB Function/1(x)
  PLL/2 -> [wt]
  Irradiance/1 -> PV Array/1
  "Temperature "/1 -> PV Array/2
  Current Measurement1/1 -> [I_Inv]
  Current Measurement/1 -> [I_Grid]
  Modulation Index/1 -> MATLAB Function/2(ma)
  PWM Generator (2-Level)/1 -> Universal Bridge/1
  Constant1/1 -> MATLAB Function/3(shift)
  Voltage Measurement1/1 -> [V_Inv]
  [V_Grid] -> PLL/1
  connections:
  Voltage Measurement1/LConn1 -- Series RLC Load/LConn1 -- Current Measurement/RConn1 -- Thyristor1/LConn1 -- Thyristor/RConn1
  Current Measurement/LConn1 -- Voltage Measurement/LConn1 -- V_Phase/RConn1
  Universal Bridge/LConn2 -- Series RLC Branch1/RConn1 -- Voltage Measurement1/LConn2 -- Series RLC Load/RConn1 -- Voltage Measurement/LConn2 -- "Neutral "/RConn1
  Thyristor/LConn1 -- Thyristor1/RConn1 -- Current Measurement1/RConn1
  Series RLC Branch3/RConn1 -- PV Array/RConn2 -- Universal Bridge/RConn2
  Series RLC Branch3/LConn1 -- PV Array/RConn1 -- Universal Bridge/RConn1
  Series RLC Branch/RConn1 -- Series RLC Branch2/LConn1 -- Series RLC Branch1/LConn1
  Series RLC Branch2/RConn1 -- Current Measurement1/LConn1
  Universal Bridge/LConn1 -- Series RLC Branch/LConn1

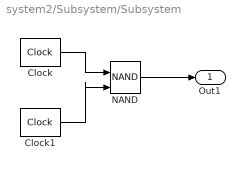
== system system2/Subsystem/Subsystem ==
  Clock : simulink_extras/Flip Flops/Clock  period=1
  Clock1 : simulink_extras/Flip Flops/Clock  period=1
  NAND : Logic  Operator=NAND  IconShape=distinctive  AllPortsSameDT=off  OutDataTypeStr=boolean
  Out1 : Outport
  wires:
  Clock/1 -> NAND/1
  Clock1/1 -> NAND/2
  NAND/1 -> Out1/1

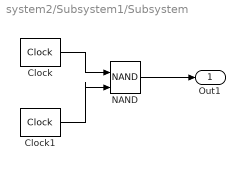
== system system2/Subsystem1/Subsystem ==
  Clock : simulink_extras/Flip Flops/Clock  period=1
  Clock1 : simulink_extras/Flip Flops/Clock  period=1
  NAND : Logic  Operator=NAND  IconShape=distinctive  AllPortsSameDT=off  OutDataTypeStr=boolean
  Out1 : Outport
  wires:
  NAND/1 -> Out1/1
  Clock1/1 -> NAND/2
  Clock/1 -> NAND/1

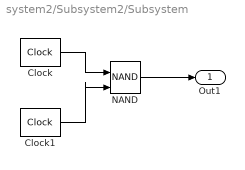
== system system2/Subsystem2/Subsystem ==
  Clock : simulink_extras/Flip Flops/Clock  period=1
  Clock1 : simulink_extras/Flip Flops/Clock  period=1
  NAND : Logic  Operator=NAND  IconShape=distinctive  AllPortsSameDT=off  OutDataTypeStr=boolean
  Out1 : Outport
  wires:
  NAND/1 -> Out1/1
  Clock1/1 -> NAND/2
  Clock/1 -> NAND/1

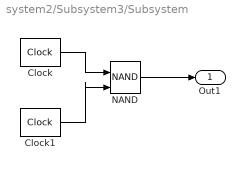
== system system2/Subsystem3/Subsystem ==
  Clock : simulink_extras/Flip Flops/Clock  period=1
  Clock1 : simulink_extras/Flip Flops/Clock  period=1
  NAND : Logic  Operator=NAND  IconShape=distinctive  AllPortsSameDT=off  OutDataTypeStr=boolean
  Out1 : Outport
  wires:
  NAND/1 -> Out1/1
  Clock1/1 -> NAND/2
  Clock/1 -> NAND/1

== matlab function system2/Subsystem/MATLAB Function ==
  data: x input; a output; ma input; shift input
function a = fcn(x,ma,shift)
shift_k = shift*(pi/180);
a = (ma*(sin((x)+shift_k)));

== matlab function system2/Subsystem2/MATLAB Function ==
  data: x input; a output; ma input; shift input
function a = fcn(x,ma,shift)
shift_k = shift*(pi/180);
a = (ma*(sin((x)+shift_k)));

== matlab function system2/Subsystem3/MATLAB Function ==
  data: x input; a output; ma input; shift input
function a = fcn(x,ma,shift)
shift_k = shift*(pi/180);
a = (ma*(sin((x)+shift_k)));

== matlab function system2/Subsystem1/MATLAB Function ==
  data: x input; a output; ma input; shift input
function a = fcn(x,ma,shift)
shift_k = shift*(pi/180);
a = (ma*(sin((x)+shift_k)));
